simulink model "AM_RXTX_Test_Sinus_Sound"  (R2020b)
settings: Solver=VariableStepAuto  StartTime=0.0  StopTime=5  RelTol=1e-3
libraries: dspsnks4 x1, dspsrcs4 x1
settings Model: Creator=Guillaume  LastModifiedBy=Guillaume

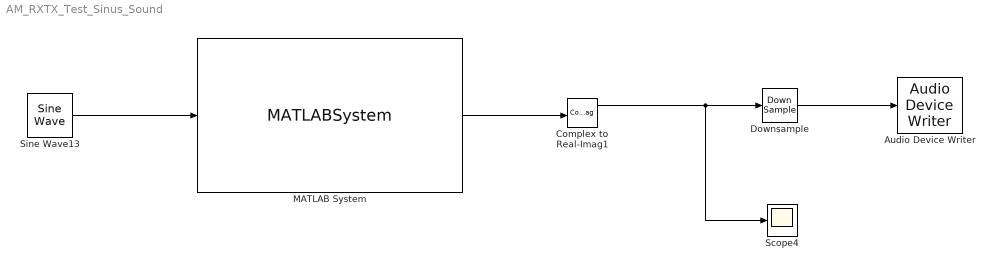
== system AM_RXTX_Test_Sinus_Sound ==
  Audio Device Writer : dspsnks4/Audio Device Writer  Driver=DirectSound  Device=Default  InheritSampleRate=on  SampleRate=44100  BitDepth=16-bit integer  BufferSize=4096  NumBuffers=10  DefaultOutputChannelMapping=on  OutputChannelMapping=1:2  OutputNumUnderrunSamples=off  DriverIdx=1  DeviceWarnFlag=''
  Complex to Real-Imag1 : ComplexToRealImag
  Downsample : DownSample  N=21  RateOptions=Allow multirate processing
  MATLAB System : MATLABSystem  System=limeSDR_Simulink_Wrapper_2022  enable_rx0=on  rx0_antenna=3  rx0_bandwidth=5  rx0_gain=20  rx_frequency=868e6  rx_samplerate=1e6  rx_timeout_ms=5000  rx_step_size=16384  enable_tx0=on  tx0_antenna=2  tx0_bandwidth=5  tx0_gain=30  tx_frequency=868e6  tx_samplerate=1e6  tx_timeout_ms=5000  tx_step_size=16384
      mask Type: limeSDR_Simulink_Wrapper_2022
      mask Display:
      | disp('LimeSDR mini');
      | port_label('input',1,'TX0 Samples');
      | port_label('output',1,'RX0 Samples');
  Scope4 : Scope
  Sine Wave13 : dspsrcs4/Sine Wave  Amplitude=1  Frequency=440  Phase=0  SampleMode=Discrete  OutComplex=Real  CompMethod=Trigonometric fcn  TableSize=Speed  SampleTime=1/1e6  SamplesPerFrame=16384  ResetState=Restart at time zero  OutputFrames=off  dataType=single  wordLen=16  udDataType=sfix(16)  fracBitsMode=Best precision  numFracBits=15  OutDataTypeStr=single  LastOutDataTypeStr=single
  wires:
  MATLAB System/1 -> Complex to Real-Imag1/1
  Downsample/1 -> Audio Device Writer/1
  Complex to Real-Imag1/1 -> Scope4/1, Downsample/1
  Sine Wave13/1 -> MATLAB System/1
